simulink library "ControllerLib"  (R2015a)
settings: Solver=ode45  StartTime=0.0  StopTime=10.0  RelTol=1e-3
libraries: vrlib x1
settings Model: Creator=tbria  LastModifiedBy=tbria

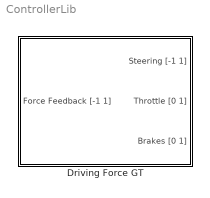
== system ControllerLib ==
  Driving Force GT : Subsystem

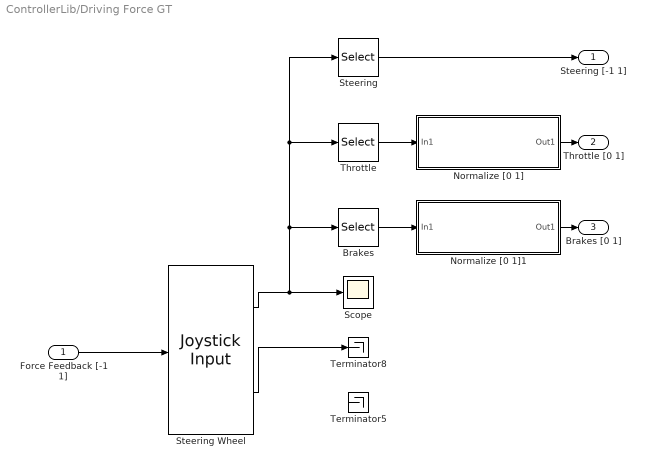
== system ControllerLib/Driving Force GT ==
  Force Feedback [-1 1] : Inport
  Brakes : Selector  InputPortWidth=4  Indices=[3]
  Normalize [0 1] : Subsystem
  Normalize [0 1]1 : Subsystem
  Scope : Scope
      settings: YMin=-0.12  YMax=0  SaveName=ScopeData16
  Steering : Selector  InputPortWidth=4  Indices=[1]
  Steering Wheel : vrlib/Joystick Input  joyid=1  adjustports=on  forcefeed=on
  Terminator5 : Terminator
  Terminator8 : Terminator
  Throttle : Selector  InputPortWidth=4  Indices=[2]
  Steering [-1 1] : Outport
  Throttle [0 1] : Outport  Port=2
  Brakes [0 1] : Outport  Port=3
  wires:
  Steering/1 -> Steering [-1 1]/1
  Normalize [0 1]1/1(Out1) -> Brakes [0 1]/1
  Normalize [0 1]/1(Out1) -> Throttle [0 1]/1
  ? -> Terminator5/1
  Steering Wheel/2 -> Terminator8/1
  Throttle/1 -> Normalize [0 1]/1(In1)
  Steering Wheel/1 -> Throttle/1, Steering/1, Brakes/1, Scope/1
  Brakes/1 -> Normalize [0 1]1/1(In1)
  Force Feedback [-1 1]/1 -> Steering Wheel/1

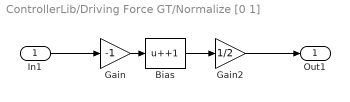
== system ControllerLib/Driving Force GT/Normalize [0 1] ==
  In1 : Inport
  Bias : Bias  Bias=+1
  Gain : Gain  Gain=-1
  Gain2 : Gain  Gain=1/2
  Out1 : Outport
  wires:
  Gain/1 -> Bias/1
  Bias/1 -> Gain2/1
  Gain2/1 -> Out1/1
  In1/1 -> Gain/1

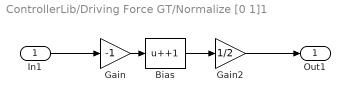
== system ControllerLib/Driving Force GT/Normalize [0 1]1 ==
  In1 : Inport
  Bias : Bias  Bias=+1
  Gain : Gain  Gain=-1
  Gain2 : Gain  Gain=1/2
  Out1 : Outport
  wires:
  Gain/1 -> Bias/1
  Bias/1 -> Gain2/1
  Gain2/1 -> Out1/1
  In1/1 -> Gain/1
